simulink model "Male_Famele"  (R2022b)
settings: Solver=VariableStepAuto  StartTime=0.0  StopTime=10.0  RelTol=1e-3
libraries: dspvision x2, audiosources x1, dspsnks4 x1
settings Model: Creator=ankas  LastModifiedBy=Carina S

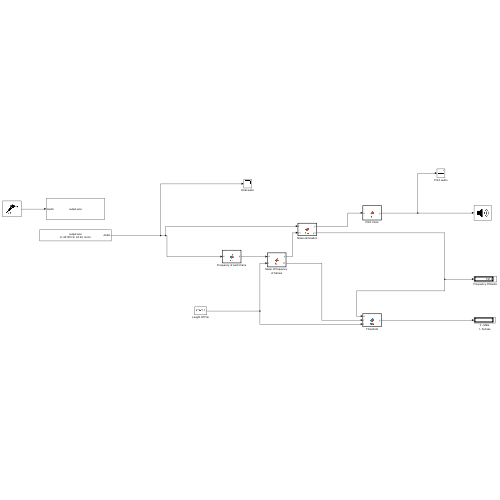
[thumbnail: Simulink's stored preview of the top-level diagram]
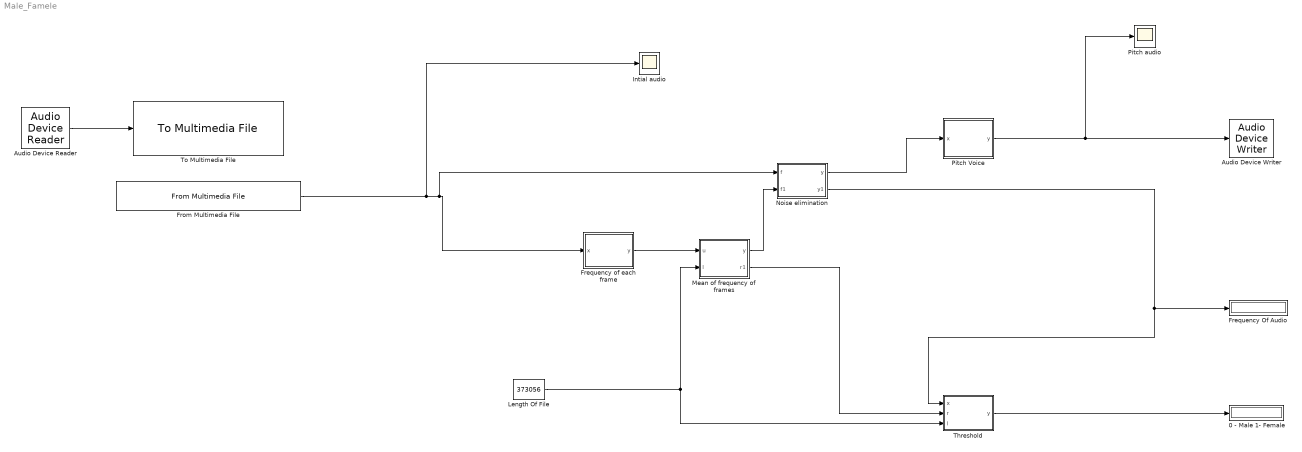
== system Male_Famele ==
  0 - Male 1- Female : Display
  Audio Device Reader : audiosources/Audio Device Reader  Driver=DirectSound  Device=Default  SampleRate=44100  NumChannels=1  SamplesPerFrame=3500  BitDepth=16-bit integer  NumBuffers=10  DefaultInputChannelMapping=on  InputChannelMapping=1:2  OutputNumOverrunSamples=off  OutputDataType=double  DriverIdx=1  DeviceWarnFlag=''
  Audio Device Writer : dspsnks4/Audio Device Writer  Driver=DirectSound  Device=Default  InheritSampleRate=on  SampleRate=44100  BitDepth=16-bit integer  BufferSize=4096  NumBuffers=10  DefaultOutputChannelMapping=on  OutputChannelMapping=1:2  OutputNumUnderrunSamples=off  DriverIdx=1  DeviceWarnFlag=''
  Frequency Of Audio : Display
  Frequency of each frame : MATLAB Function  TreatAsAtomicUnit=on
  From Multimedia File : dspvision/From Multimedia File  inputFilename=C:\Users\Carina S\Documents\Master An 1\Sem1\PMS\Proiect\output.wav  readRange=[1 Inf]  loop=on  numPlays=inf  outputStreams=Audio only  videoDataType=single  audioDataType=single  inheritSampleTime=on  userDefinedSampleTime=1/30  noAudioOutput=off  isIntensityVideo=off  fourcc=RGB  colorVideoFormat=Separate color signals  outputEOF=off  dataOrg=Column-major  audioFrameSize=3500  computeAudioFrameSize=off  outSamplingMode=Sample based
  Intial audio : Scope
  "Length Of File " : Constant  Value=373056
  Mean of frequency of frames : MATLAB Function  TreatAsAtomicUnit=on
  Noise elimination : MATLAB Function  TreatAsAtomicUnit=on
  Pitch Voice : MATLAB Function  TreatAsAtomicUnit=on
  Pitch audio : Scope
  Threshold : MATLAB Function  TreatAsAtomicUnit=on
  To Multimedia File : dspvision/To Multimedia File  outputFilename=output.wav  streamSelection=Audio only  videoCompressor=None (uncompressed)  audioCompressor=None (uncompressed)  imagePorts=Separate color signals  fileType=WAV  audioDatatype=24-bit integer  fourcc=RGB  videoQuality=75  mj2000CompFactor=10
      settings: LibrarySourceBlock=dspsnks4/To Multimedia File
  wires:
  Mean of frequency of frames/2(r1) -> Threshold/2(r)
  Threshold/1(y) -> 0 - Male 1- Female/1
  Frequency of each frame/1(y) -> Mean of frequency of frames/1(u)
  "Length Of File "/1 -> Threshold/3(l), Mean of frequency of frames/2(l)
  Noise elimination/2(y1) -> Threshold/1(x), Frequency Of Audio/1
  Mean of frequency of frames/1(y) -> Noise elimination/2(f1)
  Pitch Voice/1(y) -> Pitch audio/1, Audio Device Writer/1
  Noise elimination/1(y) -> Pitch Voice/1(x)
  From Multimedia File/1 -> Intial audio/1, Noise elimination/1(f), Frequency of each frame/1(x)
  Audio Device Reader/1 -> To Multimedia File/1

== matlab function Male_Famele/Threshold ==
  data: x input; r input; y output; l input
function y = fcn(x,r,l)
y=5;
if r>l/3500
    if x>165
        y=1;
    else
        y=0;
    end
end
end

== matlab function Male_Famele/Frequency of each frame ==
  data: x input; y output
function y = fcn(x)
Fs=44100; %frecventa de esantionare
%foloseste functia butter si filter
coder.extrinsic('butter');
coder.extrinsic('filter');
%filtru Butterworth
[b0,a0]=butter(2,325/(Fs/2));
%valoarea absoluta a semnalului de intrare
xin = abs(x);
%filtrul Butterworth aplicat pe semanlul de intrare
xin=filter(b0,a0,xin);
xin = xin-mean(xin);
x2=zeros(length(xin),1);
x2(1:length(x)-1)=xin(2:length(x));
zc=length(find((xin>0 & x2<0) | (xin<0 & x2>0)));
%frecventa undamentala
y = 0.5*Fs*zc/length(x);

== matlab function Male_Famele/Mean of frequency of frames ==
  data: u input; y output; l input; r1 output
function [ y,r1] = fcn(u,l)
persistent i
persistent r
%daca valorile lui i si r sunt goale,le intializeaza cu 0
if isempty(i)
        i = 0;
end
if isempty(r)
        r = 0;
end
j=l/3500;
i= (u/j)+i;
r=r+1;
r1=r;
y = i;

== matlab function Male_Famele/Noise elimination ==
  data: f input; y output; f1 input; y1 output
function [y, y1] = fcn(f, f1)
fs=44100;
% frecventa de taiere
fc = 2500;  
% ordinul filtrului
order = 4;
%filtrul Butterworth
[b, a] = butter(order, fc/(fs/2), 'low');  
y = filter(b, a, f);
y1=f1;

== matlab function Male_Famele/Pitch Voice ==
  data: x input; y output
function y =  f(x)
% Mărește frecvența fundamentală pentru a face vocea pitigaiata
pitchFactor = 0.6;
% Timpul pentru fiecare esantion
t_original = (0:length(x)-1)';
% Un nou vector de timp pentru esantionare
t_resampled = (0:1/pitchFactor:(length(x)-1)/pitchFactor)';
y = interp1(t_original, x, t_resampled, 'spline', 0);
end
